simulink model "Mz"  (R2024b)
settings: Solver=VariableStepAuto  StartTime=0.0  StopTime=24  RelTol=1e-3
libraries: simulink x1
settings Model: Creator=owen  LastModifiedBy=owen

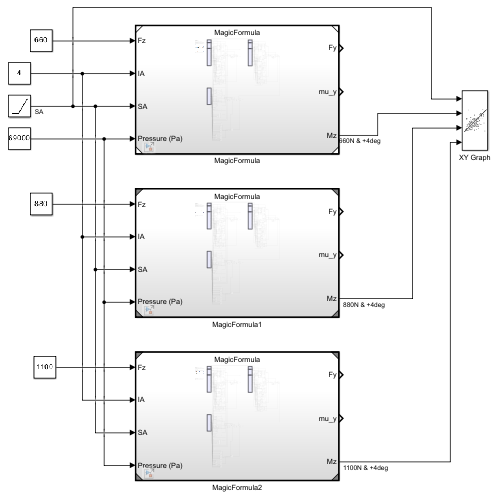
[thumbnail: Simulink's stored preview of the top-level diagram]
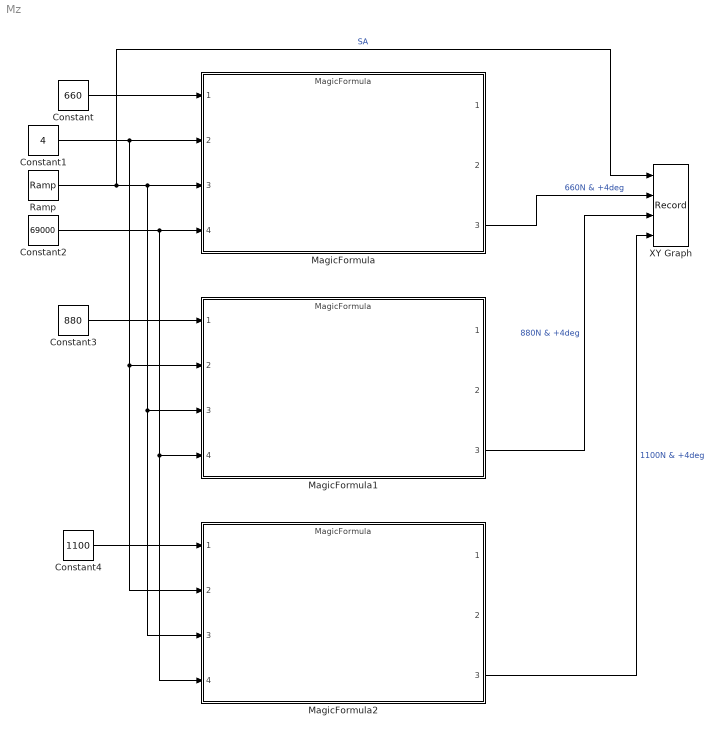
== system Mz ==
  Constant : Constant  Value=660
  Constant1 : Constant  Value=4
  Constant2 : Constant  Value=69000
  Constant3 : Constant  Value=880
  Constant4 : Constant  Value=1100
  MagicFormula : ModelReference  ModelNameDialog=MagicFormula.slx  SimulationMode=Normal  ModelReferenceVersion=1.53
  MagicFormula1 : ModelReference  ModelNameDialog=MagicFormula.slx  SimulationMode=Normal  ModelReferenceVersion=1.53
  MagicFormula2 : ModelReference  ModelNameDialog=MagicFormula.slx  SimulationMode=Normal  ModelReferenceVersion=1.53
  Ramp : simulink/Sources/Ramp  slope=1  start=0  InitialOutput=-12
  XY Graph : Record  FileSettingsInternal="{\"entries\":[{\"content\":{\"excelSettings\":{\"content\":{},\"type\":\"Streamout.ExcelSettings\"}},\"type\":\"Streamout.FileSettingStorage\",\"uuid\":\"\"}],\"packageUris\":[\"http:\\/\\/schema.mathworks.com\\/mf0\\/streamout_blocks\\/R2020a\"],\"version\":\"1.0\"}"  Layout=[1 1]  SignalsInternal="{\"entries\":[{\"content\":{\"signals\":[{\"content\":{\"blockPath\":[],\"dimensions\":[1],\"domain\":\"\",\"lineColor\":\"#ff13a6\",\"lineWidth\":2,\"port\":1,\"sid\":[\"\"],\"signalID\":1,\"signalName\":\"SA +4\"},\"type\":\"RecordBlkView.Signal\",\"uuid\":\"\"},{\"content\":{\"blockPath\":[],\"dimensions\":[1],\"domain\":\"\",\"lineColor\":\"#a2142f\",\"lineWidth\":2,\"port\":2,\"sid\":[\"\"],\"signalID\":2,\"signalName\":\"660N & +4deg\"},\"type\":\"RecordBlkView.Signal\",\"uuid\":\"\"},{\"content\":{\"blockPath\":[],\"dimensions\":[1],\"domain\":\"\",\"lineColor\":\"#22825a\",\"lineWidth\":2,\"port\":3,\"sid\":[\"\"],\"signalID\":3,\"signalName\":\"880N & +4deg\"},\"type\":\"RecordBlkView.Signal\",\"uuid\":\"\"},{\"content\":{\"blockPath\":[],\"dimensions\":[1],\"domain\":\"\",\"lineColor\":\"#00325a\",\"lineWidth\":2,\"port\":4,\"sid\":[\"\"],\"signalID\":4,\"signalName\":\"1100N & +4deg\"},\"type\":\"RecordBlkView.Signal\",\"uuid\":\"\"}]},\"type\":\"RecordBlkView.InputSignals\",\"uuid\":\"\"}],\"packageUris\":[\"http:\\/\\/schema.mathworks.com\\/mf0\\/streamout_blocks\\/R2020a\"],\"version\":\"1.0\"}"  VisualizationBindings="{\"xyplotplugin\":{\"info\":[{\"series\":[],\"subplotID\":1}]}}"  CompatibilityTag=XY
  wires:
  Constant1/1 -> MagicFormula2/2, MagicFormula1/2, MagicFormula/2
  Constant/1 -> MagicFormula/1
  Ramp/1 -> XY Graph/1, MagicFormula2/3, MagicFormula1/3, MagicFormula/3  "SA"
  Constant2/1 -> MagicFormula2/4, MagicFormula1/4, MagicFormula/4
  MagicFormula/3 -> XY Graph/2  "660N & +4deg"
  Constant3/1 -> MagicFormula1/1
  Constant4/1 -> MagicFormula2/1
  MagicFormula1/3 -> XY Graph/3  "880N & +4deg"
  MagicFormula2/3 -> XY Graph/4  "1100N & +4deg"
